simulink model "GNC_System"  (R2025b)
settings: Solver=ode45  StartTime=0.0  StopTime=150  MaxStep=0.005  RelTol=1e-3
libraries: simulink x4
settings Model: Creator=Pc  LastModifiedBy=Pc

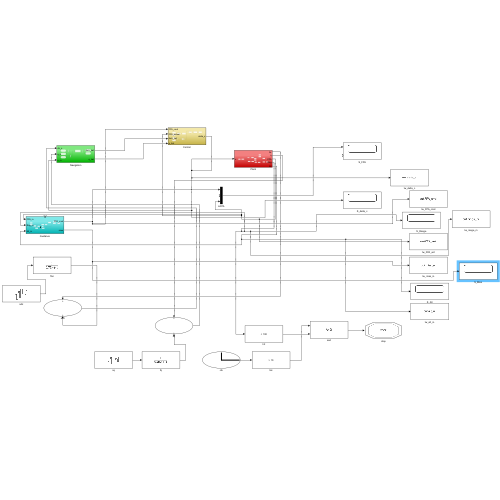
[thumbnail: Simulink's stored preview of the top-level diagram]
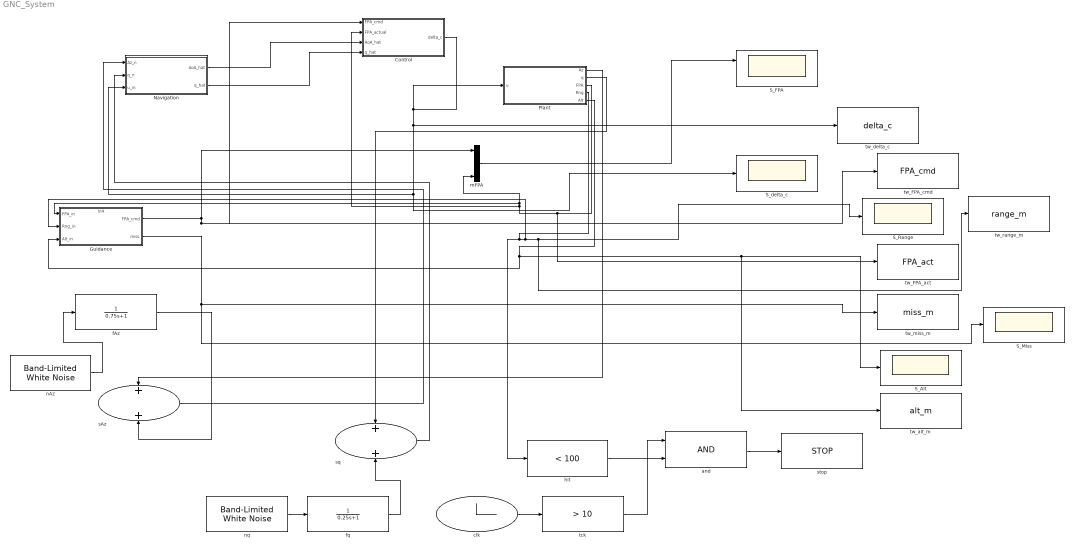
== system GNC_System ==
  Control : Subsystem
  Guidance : Subsystem
      settings: PortSchema="{\"entries\":[{\"content\":{\"sides\":[{\"content\":{\"connectorIds\":[\"In1\",\"In2\",\"In3\"]},\"type\":\"ConnectorPlacement.EquallySpacedRectSide\",\"uuid\":\"678b8a0a-00c9-4025-9ca6-704b031aac61\"},{\"content\":{\"connectorIds\":[\"Out1\",\"Out2\"],\"side\":\"RIGHT\"},\"type\":\"ConnectorPlacement.EquallySpacedRectSide\",\"uuid\":\"f7de3b39-799a-4da0-9333-6dce1b3794e6\"},{\"content\":{\"connectorIds\":[\"In4\"],\"side\":\"TOP\"},\"type\":\"ConnectorPlacement.EquallySpacedRectSide\",\"uuid\":\"84c19040-3148-4e4c-aa87-ba2c395011cd\"}]},\"type\":\"ConnectorPlacement.EquallySpacedConnector\",\"uuid\":\"8831e12e-ee3f-40f5-ad7d-507652cc4e73\"}],\"packageUris\":[\"http://schema.mathworks.com/mf0/Connector/R2020b\"],\"version\":\"1.0\"}"
  Navigation : Subsystem
  Plant : Subsystem
  S_Alt : Scope
      settings: ActiveDisplayYMinimum=212.89929761715007  ActiveDisplayYMaximum=11087.455633598094
  S_FPA : Scope  NumInputPorts=2
      settings: ActiveDisplayYMinimum=-2.96241931282787  ActiveDisplayYMaximum=-0.22889928850977703
  S_Miss : Scope
      settings: ActiveDisplayYMinimum=-10360.602550075175  ActiveDisplayYMaximum=88764.962126149461
  S_Range : Scope
      settings: ActiveDisplayYMinimum=-9660.5168000005287  ActiveDisplayYMaximum=89282.135200000048
  S_delta_c : Scope
      settings: ActiveDisplayYMinimum=-0.23223381317897265  ActiveDisplayYMaximum=0.2810408822737962
  and : Logic  AllPortsSameDT=off  OutDataTypeStr=boolean
  clk : Clock
  fAz : TransferFcn  Denominator=[0.75 1]
  fq : TransferFcn  Denominator=[0.25 1]
  hit : simulink/Logic and Bit Operations/Compare To Constant  relop=<  const=100  OutDataTypeStr=boolean
  mFPA : Mux  Inputs=3
  nAz : simulink/Sources/Band-Limited White Noise  Cov=0.55  Ts=0.01  seed=23341
  nq : simulink/Sources/Band-Limited White Noise  Cov=0.55  Ts=0.01  seed=54321
  sAz : Sum
  sq : Sum
  stop : Stop
  tck : simulink/Logic and Bit Operations/Compare To Constant  relop=>  const=10  OutDataTypeStr=boolean
  tw_FPA_act : ToWorkspace  VariableName=FPA_act  SampleTime=-1
  tw_FPA_cmd : ToWorkspace  VariableName=FPA_cmd  SampleTime=-1
  tw_alt_m : ToWorkspace  VariableName=alt_m  SampleTime=-1
  tw_delta_c : ToWorkspace  VariableName=delta_c  SampleTime=-1
  tw_miss_m : ToWorkspace  VariableName=miss_m  SampleTime=-1
  tw_range_m : ToWorkspace  VariableName=range_m  SampleTime=-1
  wires:
  nAz/1 -> fAz/1
  nq/1 -> fq/1
  Plant/1(Az) -> sAz/1
  fAz/1 -> sAz/2
  Plant/2(q) -> sq/1
  fq/1 -> sq/2
  sAz/1 -> Navigation/1(Az_n)
  sq/1 -> Navigation/2(q_n)
  Control/1(delta_c) -> S_delta_c/1, Navigation/3(u_in), tw_delta_c/1, Plant/1(u)
  Guidance/1(FPA_cmd) -> Control/1(FPA_cmd), tw_FPA_cmd/1, mFPA/1
  Plant/3(FPA) -> Guidance/1(FPA_in), mFPA/3, Control/2(FPA_actual), tw_FPA_act/1
  Navigation/1(AoA_hat) -> Control/3(AoA_hat)
  Navigation/2(q_hat) -> Control/4(q_hat)
  Plant/4(Rng) -> tw_range_m/1, S_Range/1, Guidance/2(Rng_in), hit/1
  Plant/5(Alt) -> S_Alt/1, tw_alt_m/1, Guidance/3(Alt_in)
  mFPA/1 -> S_FPA/1
  Guidance/2(miss) -> S_Miss/1, tw_miss_m/1
  clk/1 -> tck/1
  tck/1 -> and/1
  hit/1 -> and/2
  and/1 -> stop/1

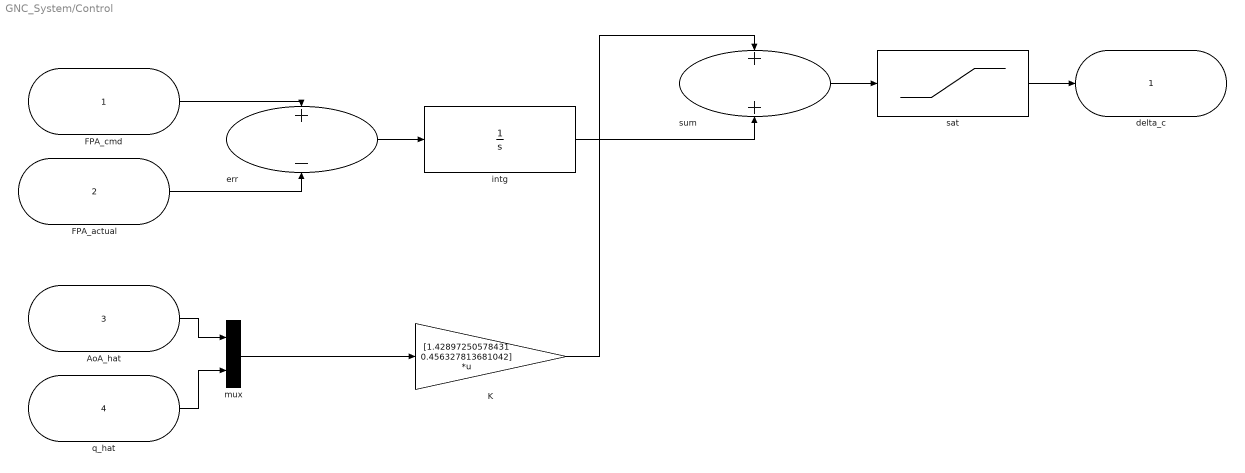
== system GNC_System/Control ==
  FPA_cmd : Inport
  FPA_actual : Inport  Port=2
  AoA_hat : Inport  Port=3
  q_hat : Inport  Port=4
  K : Gain  Gain=[1.42897250578431 0.456327813681042]  Multiplication=Matrix(K*u)
  err : Sum  Inputs=+-
  intg : Integrator  LimitOutput=on  UpperSaturationLimit=0.5  LowerSaturationLimit=-0.5
  mux : Mux  Inputs=2
  sat : Saturate  UpperLimit=0.43633  LowerLimit=-0.43633
  sum : Sum
  delta_c : Outport
  wires:
  FPA_cmd/1 -> err/1
  FPA_actual/1 -> err/2
  err/1 -> intg/1
  AoA_hat/1 -> mux/1
  q_hat/1 -> mux/2
  mux/1 -> K/1
  K/1 -> sum/1
  intg/1 -> sum/2
  sum/1 -> sat/1
  sat/1 -> delta_c/1

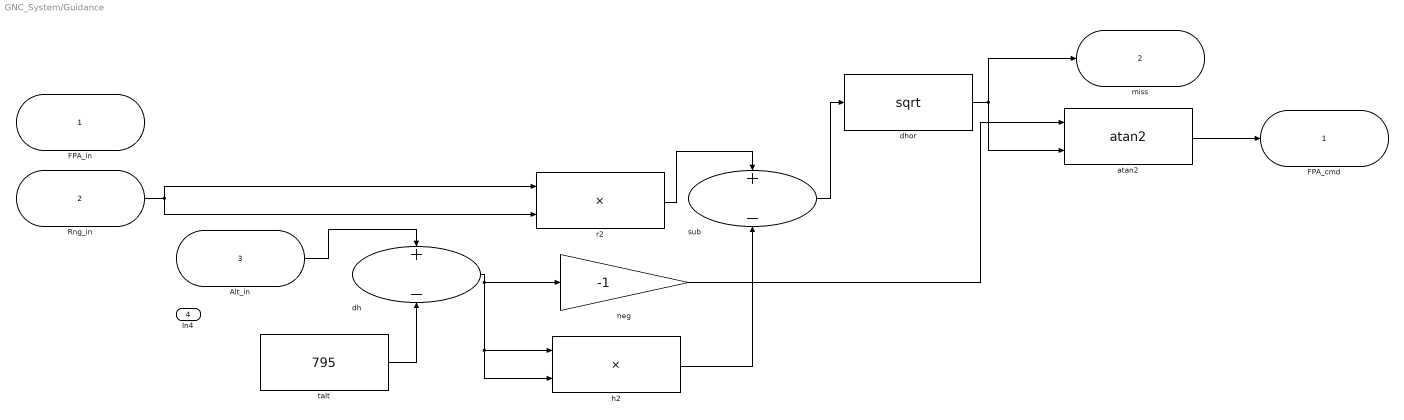
== system GNC_System/Guidance ==
  FPA_in : Inport
  Rng_in : Inport  Port=2
  Alt_in : Inport  Port=3
  In4 : Inport  Port=4
  atan2 : Trigonometry  Operator=atan2
  dh : Sum  Inputs=+-
  dhor : Math  Operator=sqrt
  h2 : Product
  neg : Gain  Gain=-1
  r2 : Product
  sub : Sum  Inputs=+-
  talt : Constant  Value=795
  FPA_cmd : Outport
  miss : Outport  Port=2
  wires:
  Alt_in/1 -> dh/1
  talt/1 -> dh/2
  Rng_in/1 -> r2/1, r2/2
  dh/1 -> h2/1, h2/2, neg/1
  r2/1 -> sub/1
  h2/1 -> sub/2
  sub/1 -> dhor/1
  neg/1 -> atan2/1
  dhor/1 -> atan2/2, miss/1
  atan2/1 -> FPA_cmd/1

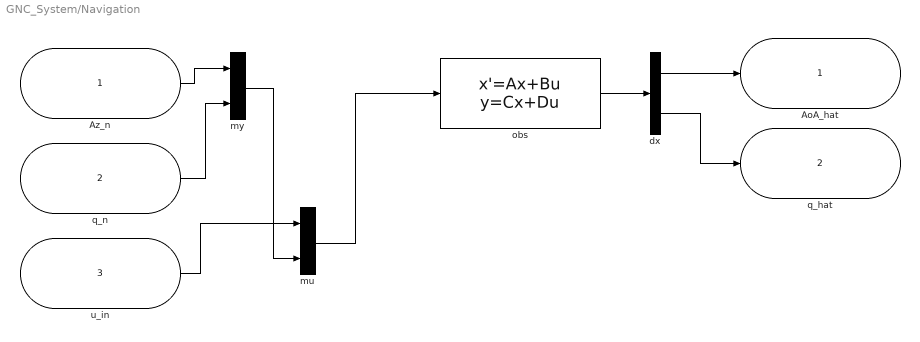
== system GNC_System/Navigation ==
  Az_n : Inport
  q_n : Inport  Port=2
  u_in : Inport  Port=3
  dx : Demux  Outputs=2
  mu : Mux  Inputs=2
  my : Mux  Inputs=2
  obs : StateSpace  A=[-33.494325 0.96260158;-278.673 -0.65848932]  B=[-0.25 -0.26293437 0.037398418;-331.4 -4.6127209 0.65848932]  C=[1 0;0 1]  D=[0 0 0;0 0 0]  InitialCondition=[0;0]
  AoA_hat : Outport
  q_hat : Outport  Port=2
  wires:
  Az_n/1 -> my/1
  q_n/1 -> my/2
  u_in/1 -> mu/1
  my/1 -> mu/2
  mu/1 -> obs/1
  obs/1 -> dx/1
  dx/1 -> AoA_hat/1
  dx/2 -> q_hat/1

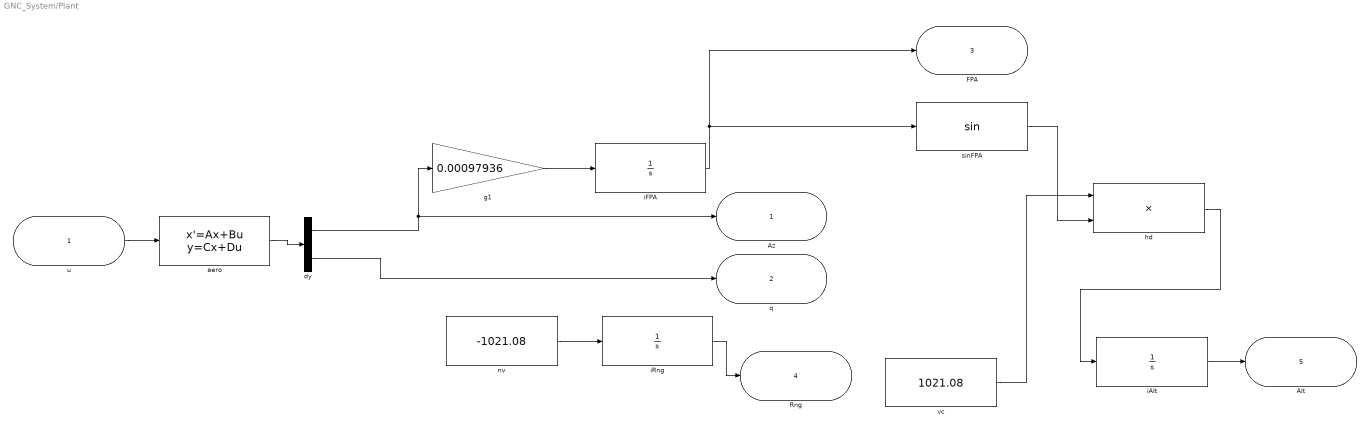
== system GNC_System/Plant ==
  u : Inport
  aero : StateSpace  A=[-1.064 1;290.26 0]  B=[-0.25;-331.4]  C=[-123.34 0;0 1]  D=[-13.51;0]  InitialCondition=[0;0]
  dy : Demux  Outputs=2
  g1 : Gain  Gain=0.00097936
  hd : Product
  iAlt : Integrator  InitialCondition=10000
  iFPA : Integrator  InitialCondition=-0.11621110
  iRng : Integrator  InitialCondition=79387.87
  nv : Constant  Value=-1021.08
  sinFPA : Trigonometry
  vc : Constant  Value=1021.08
  Az : Outport
  q : Outport  Port=2
  FPA : Outport  Port=3
  Rng : Outport  Port=4
  Alt : Outport  Port=5
  wires:
  u/1 -> aero/1
  aero/1 -> dy/1
  dy/1 -> g1/1, Az/1
  g1/1 -> iFPA/1
  nv/1 -> iRng/1
  iFPA/1 -> FPA/1, sinFPA/1
  vc/1 -> hd/1
  sinFPA/1 -> hd/2
  hd/1 -> iAlt/1
  dy/2 -> q/1
  iRng/1 -> Rng/1
  iAlt/1 -> Alt/1
